simulink model "ueb1_A1_a_ver4"  (R2016a)
settings: Solver=VariableStepAuto  StartTime=0.0  StopTime=10.0  MaxStep=0.05  RelTol=1e-3
values from neighbouring files (symbols this model uses):
  c = 10    [ueb1.m]
  d = 0.5    [ueb1.m]
  m = 1    [ueb1.m]
settings Model: Creator=bachman0  LastModifiedBy=bachman0

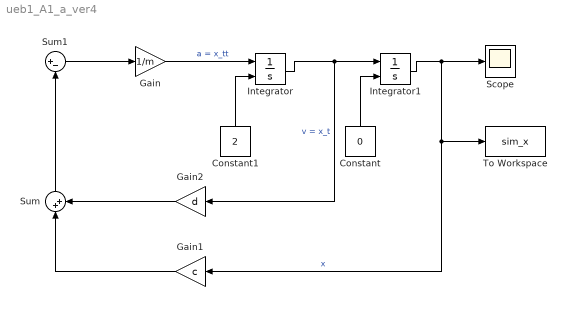
== system ueb1_A1_a_ver4 ==
  Constant : Constant  Value=0
  Constant1 : Constant  Value=2
  Gain : Gain  Gain=1/m
  Gain1 : Gain  Gain=c
  Gain2 : Gain  Gain=d
  Integrator : Integrator  InitialConditionSource=external
  Integrator1 : Integrator  InitialConditionSource=external
  Scope : Scope
  Sum : Sum  Inputs=|++
  Sum1 : Sum  Inputs=|+-
  To Workspace : ToWorkspace  VariableName=sim_x  SaveFormat=Structure With Time  SampleTime=-1
  wires:
  Integrator/1 -> Gain2/1, Integrator1/1  "v = x_t"
  Gain/1 -> Integrator/1  "a = x_tt"
  Integrator1/1 -> Scope/1, To Workspace/1, Gain1/1  "x"
  Sum1/1 -> Gain/1
  Gain1/1 -> Sum/1
  Gain2/1 -> Sum/2
  Sum/1 -> Sum1/2
  Constant/1 -> Integrator1/2
  Constant1/1 -> Integrator/2
